simulink model "dynamicmodel"  (R2017a)
settings: Solver=VariableStepAuto  StartTime=0.0  StopTime=75  RelTol=1e-3
libraries: sharedutil x6, simulink x2, aerolibutil x1
settings Model: Creator=Alex Glz  LastModifiedBy=Alex Glz

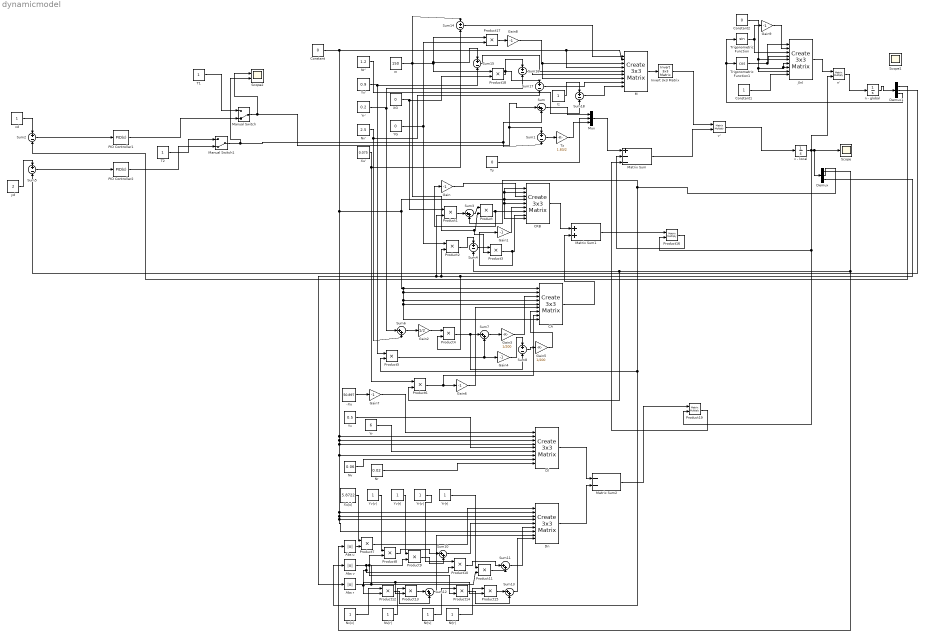
== system dynamicmodel ==
  " CRB" : sharedutil/Create 3x3 Matrix
  " J(n)" : sharedutil/Create 3x3 Matrix
  " M" : sharedutil/Create 3x3 Matrix
  -Xu : Constant  Value=50.897
  Abs r : Abs
  Abs u : Abs
  Abs v : Abs
  CA : sharedutil/Create 3x3 Matrix
  Constant : Constant  Value=0
  Constant1 : Constant
  Constant2 : Constant  Value=0
  Demux : Demux  Outputs=3
  Demux1 : Demux  Outputs=3
  Dl : sharedutil/Create 3x3 Matrix
  Dn : sharedutil/Create 3x3 Matrix
  Gain{,1,4,6..9} (7 alike) : Gain  Gain=-1
  Gain2 : Gain  Gain=1/2
  Gain3 : Gain  Gain=1/200
  Gain5 : Gain  Gain=1/200
  Invert 3x3 Matrix : aerolibutil/Invert  3x3 Matrix
  "Iz " : Constant
  Manual Switch : ManualSwitch  CurrentSetting=0
  Manual Switch1 : ManualSwitch  CurrentSetting=0
  Matrix Sum : Sum  Inputs=+--
  Matrix Sum1 : Sum
  Matrix Sum2 : Sum  Inputs=--
  Mux : Mux  Inputs=3
  Nr : Constant  Value=0.02
  Nr' : Constant  Value=1.2
  Nr|r| : Constant
  Nr|v| : Constant
  Nv : Constant  Value=0.06
  Nv' : Constant  Value=2.5
  Nv|r| : Constant
  Nv|v| : Constant
  PID Controller1 : simulink/Continuous/PID Controller  Controller=PID  TimeDomain=Continuous-time  SampleTime=-1  IntegratorMethod=Forward Euler  FilterMethod=Forward Euler  Form=Parallel  UseFilter=on  ControllerParametersSource=internal  P=2  I=0  D=2  N=100  InitialConditionSource=internal  InitialConditionForIntegrator=0  InitialConditionForFilter=0  ExternalReset=none  LimitOutput=off  UpperSaturationLimit=inf  LowerSaturationLimit=-inf  LinearizeAsGain=on  AntiWindupMode=none  Kb=1  TrackingMode=off  Kt=1  PParamMin=[]  PParamMax=[]  IParamMin=[]  IParamMax=[]  DParamMin=[]  DParamMax=[]  NParamMin=[]  NParamMax=[]  KbParamMin=[]  KbParamMax=[]  KtParamMin=[]  KtParamMax=[]  POutMin=[]  POutMax=[]  IOutMin=[]  IOutMax=[]  DOutMin=[]  DOutMax=[]  NOutMin=[]  NOutMax=[]  KbOutMin=[]  KbOutMax=[]  KtOutMin=[]  KtOutMax=[]  IntegratorOutMin=[]  IntegratorOutMax=[]  FilterOutMin=[]  FilterOutMax=[]  SumOutMin=[]  SumOutMax=[]  SumI1OutMin=[]  SumI1OutMax=[]  SumI2OutMin=[]  SumI2OutMax=[]  SumI3OutMin=[]  SumI3OutMax=[]  SumDOutMin=[]  SumDOutMax=[]  SaturationOutMin=[]  SaturationOutMax=[]  IntegratorContinuousStateAttributes=''  IntegratorStateMustResolveToSignalObject=off  IntegratorRTWStateStorageClass=Auto  FilterContinuousStateAttributes=''  FilterStateMustResolveToSignalObject=off  FilterRTWStateStorageClass=Auto  DifferentiatorICPrevScaledInput=0  DifferentiatorOutMin=[]  DifferentiatorOutMax=[]  InitialConditionSetting=State (most efficient)
  PID Controller2 : simulink/Continuous/PID Controller  Controller=PID  TimeDomain=Continuous-time  SampleTime=-1  IntegratorMethod=Forward Euler  FilterMethod=Forward Euler  Form=Parallel  UseFilter=on  ControllerParametersSource=internal  P=2  I=0  D=2  N=100  InitialConditionSource=internal  InitialConditionForIntegrator=0  InitialConditionForFilter=0  ExternalReset=none  LimitOutput=off  UpperSaturationLimit=inf  LowerSaturationLimit=-inf  LinearizeAsGain=on  AntiWindupMode=none  Kb=1  TrackingMode=off  Kt=1  PParamMin=[]  PParamMax=[]  IParamMin=[]  IParamMax=[]  DParamMin=[]  DParamMax=[]  NParamMin=[]  NParamMax=[]  KbParamMin=[]  KbParamMax=[]  KtParamMin=[]  KtParamMax=[]  POutMin=[]  POutMax=[]  IOutMin=[]  IOutMax=[]  DOutMin=[]  DOutMax=[]  NOutMin=[]  NOutMax=[]  KbOutMin=[]  KbOutMax=[]  KtOutMin=[]  KtOutMax=[]  IntegratorOutMin=[]  IntegratorOutMax=[]  FilterOutMin=[]  FilterOutMax=[]  SumOutMin=[]  SumOutMax=[]  SumI1OutMin=[]  SumI1OutMax=[]  SumI2OutMin=[]  SumI2OutMax=[]  SumI3OutMin=[]  SumI3OutMax=[]  SumDOutMin=[]  SumDOutMax=[]  SaturationOutMin=[]  SaturationOutMax=[]  IntegratorContinuousStateAttributes=''  IntegratorStateMustResolveToSignalObject=off  IntegratorRTWStateStorageClass=Auto  FilterContinuousStateAttributes=''  FilterStateMustResolveToSignalObject=off  FilterRTWStateStorageClass=Auto  DifferentiatorICPrevScaledInput=0  DifferentiatorOutMin=[]  DifferentiatorOutMax=[]  InitialConditionSetting=State (most efficient)
  Product{,1..15,17..18} (18 alike) : Product
  Product16 : Product  Multiplication=Matrix(*)
  Product19 : Product  Multiplication=Matrix(*)
  Scope : Scope
  Scope1 : Scope
  Scope2 : Scope  NumInputPorts=2
  Sum{,3,6..7,10..13} (8 alike) : Sum  Inputs=|++
  Sum{1..2,4..5,8,14..18} (10 alike) : Sum  Inputs=+-
  T1 : Constant
  T2 : Constant
  Trigonometric Function : Trigonometry
  Trigonometric Function1 : Trigonometry  Operator=cos
  Ty : Constant  Value=0
  Tz : Gain  Gain=1.83/2
  XG : Constant  Value=0
  Xu' : Constant  Value=0.075
  Xu|u| : Constant  Value=5.8722
  YG : Constant  Value=0
  Yr : Constant  Value=6
  Yr' : Constant  Value=0.2
  Yr|r| : Constant
  Yr|v| : Constant
  Yv : Constant  Value=0.5
  Yv' : Constant  Value=0.9
  Yv|r| : Constant
  Yv|v| : Constant
  m : Constant  Value=150
  n - global : Integrator  InitialCondition=[0 0 .3]
  n' : Product  Multiplication=Matrix(*)
  v - local : Integrator
  v' : Product  Multiplication=Matrix(*)
  xd : Constant
  yd : Constant  Value=2
  wires:
  Manual Switch/1 -> Scope2/1, Sum/1, Sum1/1
  Manual Switch1/1 -> Scope2/2, Sum/2, Sum1/2
  Sum1/1 -> Tz/1
  Sum/1 -> Mux/1
  Ty/1 -> Mux/2
  Tz/1 -> Mux/3
  Mux/1 -> Matrix Sum/1
  Sum3/1 -> Product/1
  Product1/1 -> Sum3/1
  XG/1 -> Product18/2, Product1/1
  m/1 -> Product18/1, Sum15/1, Product17/1, Product3/2, Product/2, Sum14/1
  Product2/1 -> Sum4/1
  YG/1 -> Product17/2, Product2/1
  Sum4/1 -> Product3/1
  Product/1 -> Gain/1, " CRB"/7
  Product3/1 -> Gain1/1, " CRB"/8
  Gain/1 -> " CRB"/3
  Gain1/1 -> " CRB"/6
  " CRB"/1 -> Matrix Sum1/1
  CA/1 -> Matrix Sum1/2
  Matrix Sum1/1 -> Product16/1
  v - local/1 -> n'/2, Product19/2, Product16/2, Demux/1, Scope/1
  Demux/1 -> Abs u/1, Product6/2, Sum4/2
  Demux/2 -> Sum3/2, Abs v/1, Product5/2
  Demux/3 -> Abs r/1, Product1/2, Product2/2, Product4/2
  Gain2/1 -> Product4/1
  Sum6/1 -> Gain2/1
  Yr'/1 -> Sum16/2, Sum6/1
  Nv'/1 -> Sum17/2, Sum6/2
  Yv'/1 -> Sum15/2, Product5/1
  Product4/1 -> Sum8/2, Sum7/1
  Product5/1 -> Gain4/1, Sum7/2
  Sum7/1 -> Gain3/1
  Gain3/1 -> CA/3
  Sum8/1 -> Gain5/1
  Gain4/1 -> Sum8/1
  Gain5/1 -> CA/7
  Xu'/1 -> Sum14/2, Product6/1
  Product6/1 -> CA/8, Gain6/1
  Gain6/1 -> CA/6
  Dl/1 -> Matrix Sum2/1
  Dn/1 -> Matrix Sum2/2
  Matrix Sum2/1 -> Product19/1
  Constant/1 -> " M"/4, " M"/2, Dn/3, Dn/4, Dn/7, Dn/2, Dl/7, Dl/4, Dl/3, Dl/2, " CRB"/2, " CRB"/1, " CRB"/9, " CRB"/5, " CRB"/4, CA/9, CA/5, CA/4, CA/2, CA/1
  -Xu/1 -> Gain7/1
  Gain7/1 -> Dl/1
  Yv/1 -> Dl/5
  Yr/1 -> Dl/6
  Nv/1 -> Dl/8
  Nr/1 -> Dl/9
  Xu|u|/1 -> Product7/1
  Abs u/1 -> Product7/2
  Product7/1 -> Dn/1
  Yv|v|/1 -> Product8/1
  Abs v/1 -> Product15/2, Product13/2, Product12/2, Product10/2, Product14/2, Product8/2
  Yv|r|/1 -> Product9/1
  Abs r/1 -> Product11/2, Product9/2
  Product8/1 -> Sum10/1
  Product9/1 -> Sum10/2
  Sum10/1 -> Dn/5
  Product11/1 -> Sum11/2
  Product10/1 -> Sum11/1
  Yr|v|/1 -> Product10/1
  Yr|r|/1 -> Product11/1
  Sum11/1 -> Dn/6
  Sum12/1 -> Dn/8
  Sum13/1 -> Dn/9
  Product15/1 -> Sum13/1
  Product14/1 -> Sum13/2
  Product13/1 -> Sum12/1
  Product12/1 -> Sum12/2
  Nv|v|/1 -> Product12/1
  Nv|r|/1 -> Product13/1
  Nr|v|/1 -> Product14/1
  Nr|r|/1 -> Product15/1
  Matrix Sum/1 -> v'/2
  " M"/1 -> Invert 3x3 Matrix/1
  v'/1 -> v - local/1
  Sum14/1 -> " M"/1
  Product17/1 -> Gain8/1
  Gain8/1 -> " M"/7, " M"/3
  Sum15/1 -> " M"/5
  Product18/1 -> Sum17/1, Sum16/1
  Sum16/1 -> " M"/6
  Sum17/1 -> " M"/8
  "Iz "/1 -> Sum18/1
  Nr'/1 -> Sum18/2
  Sum18/1 -> " M"/9
  Invert 3x3 Matrix/1 -> v'/1
  Product16/1 -> Matrix Sum/2
  Product19/1 -> Matrix Sum/3
  Trigonometric Function/1 -> " J(n)"/3, Gain9/1
  Gain9/1 -> " J(n)"/2
  Trigonometric Function1/1 -> " J(n)"/4, " J(n)"/1
  Constant1/1 -> " J(n)"/9
  Constant2/1 -> " J(n)"/8, " J(n)"/7, " J(n)"/6, " J(n)"/5
  n - global/1 -> Demux1/1
  Demux1/3 -> Trigonometric Function/1, Trigonometric Function1/1
  n'/1 -> n - global/1
  " J(n)"/1 -> n'/1
  T1/1 -> Manual Switch/1
  PID Controller1/1 -> Manual Switch/2
  T2/1 -> Manual Switch1/1
  PID Controller2/1 -> Manual Switch1/2
  xd/1 -> Sum2/1
  yd/1 -> Sum5/1
  Demux1/1 -> Sum2/2
  Demux1/2 -> Sum5/2
  Sum5/1 -> PID Controller2/1
  Sum2/1 -> PID Controller1/1
